simulink model "BasicAudio_TranslationEngine64"  (R2022b)
settings: Solver=FixedStepDiscrete  StartTime=0.0  StopTime=5  RelTol=1e-3  EnableMultiTasking=on
InitFcn:
  | % Initialize model
  | run([ ModelRootName() 'Init.m' ]);
  | 
  | % load library data
  | GainLibrary_data;
  | % Load saved values from partition process
  | CapturedConstMask.LoadMapFromFile(bdroot)
model workspace (MAT data in the model file):
  PreampVolumeTable_Idx = Simulink.Signal
  PreampVolumeTable_Idx.DataType = 'auto'
  PreampVolumeTable_Idx.Dimensions = -1
  PreampVolumeTable_Idx.DimensionsMode = 'auto'
  PreampVolumeTable_Idx.Complexity = 'auto'
  PreampVolumeTable_Idx.SampleTime = -1
  PreampVolumeTable_Idx.SamplingMode = 'auto'
  PreampVolumeTable_Idx.InitialValue = 'uint8([0 255 255 255 255 255])'
  Range = Simulink.Signal
  Range.DataType = 'auto'
  Range.Dimensions = -1
  Range.DimensionsMode = 'auto'
  Range.Complexity = 'auto'
  Range.SampleTime = -1
  Range.SamplingMode = 'auto'
  Table_Idx = Simulink.Signal
  Table_Idx.DataType = 'auto'
  Table_Idx.Dimensions = -1
  Table_Idx.DimensionsMode = 'auto'
  Table_Idx.Complexity = 'auto'
  Table_Idx.SampleTime = -1
  Table_Idx.SamplingMode = 'auto'
undefined symbols (not defined in the file or in its folder): Row
libraries: TuneVar x50, TOP x27, FeaturePath x7, CapturedConstLib x3
(part 1 of 4)
settings Model: Creator=kl13806
settings DataIOCC: ReturnWorkspaceOutputs=off
settings OptimizationCC: DefaultParameterBehavior=Inlined  DefaultUnderspecifiedDataType=single  EfficientTunableParamExpr=on
settings DebuggingCC: MergeDetectMultiDrivingBlocksExec=none  InheritedTsInSrcMsg=none  MultiTaskDSMMsg=none  ParameterPrecisionLossMsg=none  ParameterTunabilityLossMsg=error  UnconnectedInputMsg=warning  UnconnectedOutputMsg=warning  UnconnectedLineMsg=warning  UnknownTsInhSupMsg=none  SFUnexpectedBacktrackingDiag=warning  SFNoUnconditionalDefaultTransitionDiag=warning  SFExecutionAtInitializationDiag=none  SFMachineParentedDataDiag=warning
settings HardwareCC: ProdBitPerPointer=32  ProdBitPerSizeT=32  ProdBitPerPtrDiffT=32  ProdWordSize=32  ProdHWDeviceType=Intel->x86-32 (Windows32)  TargetBitPerPointer=64  TargetBitPerSizeT=64  TargetBitPerPtrDiffT=64  TargetLongLongMode=on  TargetIntDivRoundTo=Zero  TargetEndianess=LittleEndian  TargetWordSize=64  TargetHWDeviceType=MATLAB Host  ProdEqTarget=off
settings ModelReferenceCC: EnableRefExpFcnMdlSchedulingChecks=on  ModelReferenceNumInstancesAllowed=Single
settings SFSimCC: MATLABDynamicMemAlloc=off
settings RTWCC: Description=Embedded Coder (host-based shared library target)  SystemTargetFile=ert_shrlib.tlc  TLCOptions="-aTALARIA_ENGINE=\"Translation\""  TemplateMakefile=ert_default_tmf  RTWVerbose=off  RetainRTWFile=on  Toolchain=MinGW64 | gmake (64-bit Windows)  IncludeHyperlinkInReport=on
settings RTWCC: CustomHeaderCode=|
  | // Auto-generated code for model BasicAudio
  | /**** TOP TOKEN COMPATIBILITY HASH VALUES ****/
  | #define TOP_COMPAT {0x6E521A79UL}
  | #define TOP_COMPAT_NAME {"BasicAudio"}
  | #define TOP_COMPAT_NAME_HASH {0x9FD22631UL}
  | /**** COMPAT HASH VALUES BY MODULE ****/
  | #define BASICAUDIO_TOP_COMPAT 0x6E521A79UL
  | /**** NAME HASH VALUES BY MODULE ****/
  | #define BASICAUDIO_TOP_NAME_HASH 0x9FD22631UL
settings CodeAppCC: ForceParamTrailComments=on  IgnoreCustomStorageClasses=off  MaxIdLength=128  OperatorAnnotations=on  SimulinkDataObjDesc=on  SFDataObjDesc=on  MATLABFcnDesc=on  InsertBlockDesc=on  StateflowObjectComments=on  MATLABSourceComments=on
settings STFCustomTargetCC: TargetLangStandard=C99 (ISO)  MultiwordLength=256  ParMdlRefBuildCompliant=on  CompOptLevelCompliant=on  CombineOutputUpdateFcns=on  ERTCustomFileBanners=on  SupportContinuousTime=off  SupportNonInlinedSFcns=off  RemoveResetFunc=on  SupportVariableSizeSignals=on  MATLABClassNameForMDSCustomization=Simulink.SoftwareTarget.ERTCustomization  ModelStepFunctionPrototypeControlCompliant=on  UseToolchainInfoCompliant=on  SystemTargetFile=ert_shrlib.tlc
settings ERTTargetCC: TargetLangStandard=C99 (ISO)  ConcurrentExecutionCompliant=off  SupportVariableSizeSignals=on  CPPClassGenCompliant=off  InlinedParameterPlacement=NonHierarchical  ERTCustomFileTemplate=translation_dll.tlc  IndentStyle=Allman  IndentSize=4

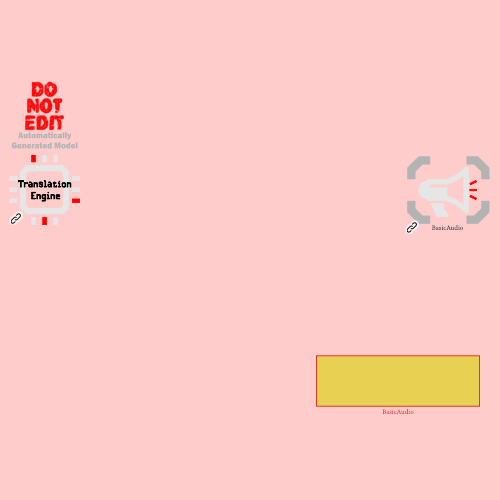
[thumbnail: Simulink's stored preview of the top-level diagram]
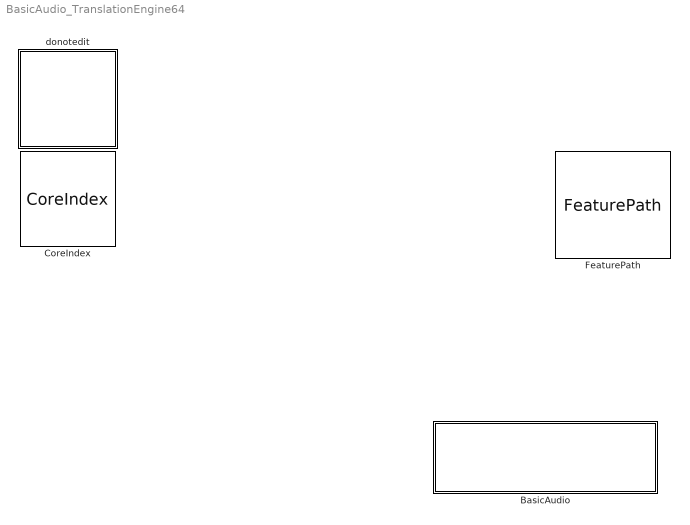
== system BasicAudio_TranslationEngine64 ==
  BasicAudio : Subsystem
  CoreIndex : FeaturePath/CoreIndex  Role=Translation Engine  CoreIndex=9  Config=[]  AddressingMode=Directly include core number in message identifiers (i.e. simple and static)  CrossCoreApi=FourListChipManager  CrossCoreAllocation=LocalCore  CrossCoreSampleTime=-1  BasePeriod=[]  TriggerInit=[-490 -501 -395 -406]
      settings: SourceProductName=Bose Talaria
  FeaturePath : FeaturePath/FeaturePath  FeatureName=BasicAudio  IsGroup=on  GroupNumber=-1  IsModule=off  TriggerInit=[45 -501 160 -394]
      settings: SourceProductName=Bose Talaria
  donotedit : Subsystem
      settings: OpenFcn=BasicAudio
      mask Display: image('DoNotEdit.svg');

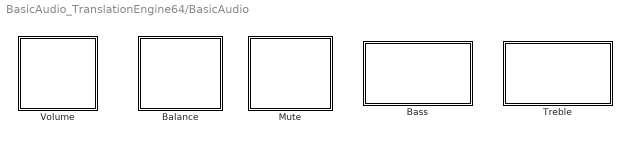
== system BasicAudio_TranslationEngine64/BasicAudio ==
  Balance : Subsystem  TreatAsAtomicUnit=on
  Bass : Subsystem  TreatAsAtomicUnit=on
  Mute : Subsystem  TreatAsAtomicUnit=on
  Treble : Subsystem  TreatAsAtomicUnit=on
  Volume : Subsystem  TreatAsAtomicUnit=on

== system BasicAudio_TranslationEngine64/donotedit ==

== system BasicAudio_TranslationEngine64/BasicAudio/Balance ==
  balance : Subsystem  mask(Bose Audio Balance){MaskFeatureName=Balance, MaskOffset=127, MaskChanRampMap=[1  2], BankNumber=0, MaskSilentExtreme=off, MaskSilentExtremeBass=on, MaskBoostDisable=off}
      mask prompts: MaskFeatureName "Feature Name (controls FeaturePath)"; MaskOffset "Control index offset"; MaskChanRampMap "Channel to Ramper map"; BankNumber "Target memory bank number:"; MaskSilentExtreme "Enable silent extreme"; MaskSilentExtremeBass "Enable silent extreme mutes bass"; MaskBoostDisable "Disable boost"
      mask help:
      | This Balance block allows for runtime control of balancing between left and right speakers/content. Based on a gain index which comes in through a control message, channel gains for 4 different content types are computed: Left, Right, Center, and Mono.
      |
      | For the Channel to Ramper Map, enter any of the following values:
      | 1 - left channel
      | 2 - right channel
      | 3 - center channel
      | 4 - mono channel
      | -1 - unused channel (will esentially be muted)
      |
      | Enable Silent Extreme if the desired outcome when accepting an index of 0 (hard left) or 255 (hard right) should completely mute the opposing channel.
      |
      | If Silent Extreme Mutes Bass is enabled, then all mono channels will be muted, when Silent Extreme is activated.
      |
      | If this block is being used in conjunction with a stand-alone Sleeping Beauty block, disable the two Silent Extreme options.
      mask init:
      | blkh = gcbh;
      | % Copy discrete mask parameters into a classdef object
      | InnerLinkConfig = BalanceConfig;
      | InnerLinkConfig.DefaultMaskOffset = MaskOffset;
      | InnerLinkConfig.DefaultMaskChanRampMap = MaskChanRampMap;
      | InnerLinkConfig.BankNumber = BankNumber;
      | InnerLinkConfig.DefaultMaskSilentExtreme = MaskSilentExtreme;
      | InnerLinkConfig.DefaultMaskSilentExtremeBass = MaskSilentExtremeBass;
      | InnerLinkConfig.DefaultMaskBoostDisable = MaskBoostDisable;
      mask Help:
      | The Balance block includes runtime control support for adjusting the balance dynamically.
      | - Channels may to be assigned to one of 4 possible rampers. Each channel needs to be assigned to a valid ramper (i.e. 1 - 4, or -1 for unused).
      | - The Index offset determines the index which corresponds to the balance being in the center position (typically 128).
      | - 'Enable silent extreme' mutes the speakers of the group whose gains are being 'cut' when at extreme indices.
      | - 'Disable boost' determines whether a boost is required or not. If selected, the maximum boost will be '1' on the linear scale ('0' in dB), otherwise he boost is calculated based on the curve (typically a maximum of 3 dB).
      | 
      | Control messages can be sent through the RTC block. The block is configured to accept a ramp time or rate (the rate has precedence) and an index which determines the gains for each channel group.
      | E.g., RTC_SIM_OBJ.AddREQ( 'BalanceSet', 0.1, [0001, <balance_index>, <ramp_db_per_second>, <ramp_milliseconds>, <subwoofer_index>, <surround_volume_index>]);
      | E.g., RTC_SIM_OBJ.AddREQ( 'BalanceSet', 0.1, [0001, 255, 0, 50, 128, 192]);
      mask TypeOptions MaskFeatureName: InnerLink/FeatureName
      mask Display:
      | [path,w,h] = IconBalanceMask();
      | 
      | % work in pixels since the icon does not scale
      | pos = get(gcbh,'position');
      | bw = pos(3) - pos(1);
      | bh = pos(4) - pos(2);
      | 
      | % Draw centered icon
      | xAdj = bw/2 - w/2;
      | yAdj = bh/2 - h/2;
      | for i=1:length(path)
      |     if (path(i).rgb(1) >= 0)
      |         patch(path(i).x+xAdj, path(i).y+yAdj, path(i).rgb);
      |     end
      |     if (path(i).stroke(1) >= 0)
      |         plot(path(i).x+xAdj, path(i).y+yAdj);
      |     end
      | end
      | 
      | % place feature name text
      | text(bw*0.5, 0, [MaskFeatureName '\n\n'], 'horizontalAlignment', 'center');

== system BasicAudio_TranslationEngine64/BasicAudio/Bass ==
  Tone : Subsystem  mask(Bose Tone High/Low){MaskFeatureName=Bass, MaskFilterType=lowpass, MaskCutHz=200, MaskCut_dB=20, MaskBoostHz=200, MaskBoost_dB=20, MaskDefaultOffset=128, MaskDefaultScale=127, BankNumber=0, TriggerInit=[90 20 195 80]}
      mask prompts: MaskFeatureName "Tone Filter Name (controls FeaturePath)"; MaskFilterType "Filter Type"; MaskCutHz "Cutoff Hz"; MaskCut_dB "Maximum dB"; MaskBoostHz "Cutoff Hz"; MaskBoost_dB "Maximum dB"; MaskDefaultOffset "Default Offset"; MaskDefaultScale "Default Scale"; BankNumber "Memory Bank Number:"; TriggerInit "Hidden: MoveFcn redraw"
      mask help: The tone block performs the treble and bass tone controls across multiple channels via a 1st order filter.
      mask init:
      | blkh = gcbh;
      | % Copy discrete mask parameters into a classdef object
      | InnerLinkConfig = ToneConfig;
      | InnerLinkConfig.FilterType = MaskFilterType;
      | InnerLinkConfig.DefaultCutHz = MaskCutHz;
      | InnerLinkConfig.DefaultCutDb = MaskCut_dB;
      | InnerLinkConfig.DefaultBoostHz = MaskBoostHz;
      | InnerLinkConfig.DefaultBoostDb = MaskBoost_dB;
      | InnerLinkConfig.DefaultOffset = MaskDefaultOffset;
      | InnerLinkConfig.DefaultScale = MaskDefaultScale;
      | InnerLinkConfig.BankNumber = BankNumber;
      settings: MoveFcn=toneMask.CB_TriggerInit(gcbh);
      mask Help:
      | The tone block performs the treble and bass tone controls across multiple channels via a 1st order filter. The treble/ bass content can either be 'boosted' or 'cut' depending on the value of the gain. Different filters can be used for the boost and cut regions, each with its own cut-off frequency.
      | 
      | MASK PARAMETERS:
      | - Different filter coefficients can be applied for the boost and cut regions
      | - The maximum boost/ cut can be specified (typically 20 dB and -20 dB)
      | - The offset and scale values determine the piecewise linear curve that maps the index to the gain (typically 128 and 127 respectively)
      | 
      | RTC CONTROL:
      | Run time control is available to dynamically change the gain to be applied to the treble/bass content. An index (typically between 0-255) can be provided along with a ramp time and rate (rate gets precedence).
      | RTC_SIM_OBJ.AddREQ( 'TrebleBassSet', 0.6, [0005,  <tone_index>, <ramp_db_per_second>, <ramp_time>]);
      | E.g., RTC_SIM_OBJ.AddREQ( 'TrebleBassSet', 0.6, [0005,  50, 0, 50]);
      mask TypeOptions MaskFeatureName: InnerLink/FeatureName
      mask TypeOptions MaskFilterType: lowpass | highpass
      mask Callback TriggerInit: ToneMask.CB_TriggerInit(gcbh);
      mask DialogControl GroupFilter Prompt: ToneFilter
      mask DialogControl GroupCut Prompt: Cut Filter
      mask DialogControl GroupBoost Prompt: Boost Filter
      mask DialogControl CalibrationGroup Prompt: Control Signal Calibration
      mask DialogControl CalibText Prompt:
      | Set the Offset and Scale to normalize the input value between -1 (maximum cut) and 1 (maximum boost) so the following equation becomes true:
      | 
      | normalized-float-value = (integer-RTC-value + Offset)  * Scale
      mask Display:
      | [path w h] = IconToneMask();
      | 
      | % retrieve the block's pixel size
      | pos = get(gcbh,'position');
      | bw = pos(3) - pos(1);
      | bh = pos(4) - pos(2);
      | 
      | % draw centered icon
      | xAdj = bw/2 - w/2;
      | yAdj = bh/2 - h/2 + 4;
      | for i=1:length(path)
      | 	patch(path(i).x+xAdj, path(i).y+yAdj, path(i).rgb);
      | end
      | 
      | % place feature name text
      | 	text(bw*0.5, 0, [MaskFeatureName '\n\n'], 'horizontalAlignment', 'center');
      | 
      | % retrieve the block's pixel size
      | pos = get(gcbh,'position');
      | bw = pos(3) - pos(1);
      | bh = pos(4) - pos(2);

== system BasicAudio_TranslationEngine64/BasicAudio/Mute ==
  mute : Subsystem  mask(Bose Audio Mute){initial_mute_state=0, MaskFeatureName=Mute, samplesPerFrame=32}
      mask prompts: initial_mute_state "Initially muted (logical)"; MaskFeatureName "Feature Name"; samplesPerFrame "Samples per frame"
      mask help: This block offers a simple mute feature using rgainy block. Set initial mute state for system cold start and a feature path name as desired. There are no tunable components, but runtime control is included.
      mask init:
      | blkh = gcbh;
      | % Copy discrete mask parameters into a classdef object
      | InnerLinkConfig = MuteConfig;
      | InnerLinkConfig.InitialMuteState = initial_mute_state;
      | InnerLinkConfig.SamplesPerFrame = samplesPerFrame;
      | 
      | % Support icon display use of ok
      | [ok,found] = MaskUtil.GetEvaluatedParameter(...
      |     MaskUtil.SubBlockName(blkh,'InnerLink'),'ok');
      | if (found == false)
      |     ok = true;
      | end
      mask Help:
      | This block offers a simple mute feature using rgainy block. The initial mute status of the block can be set through the mask.
      | 
      | RTC CONTROL:
      | Run time control is available to dynamically mute the audio. The mute status can be provided ('1' to mute audio), along with a ramp time and rate (rate gets precedence).
      | RTC_SIM_OBJ.AddREQ( 'MuteSet', 0.6, [0005,  <mute_status>, <ramp_db_per_second>, <ramp_time>]);
      | E.g., RTC_SIM_OBJ.AddREQ( 'MuteSet', 0.7, [0002, 1, 0, 50]);
      mask TypeOptions MaskFeatureName: InnerLink/FeatureName
      mask Display:
      | [path,w,h] = IconMuteMask();
      | 
      | % work in pixels since the icon does not scale
      | pos = get(gcbh,'position');
      | bw = pos(3) - pos(1);
      | bh = pos(4) - pos(2);
      | 
      | % Draw centered icon
      | xAdj = bw/2 - w/2;
      | yAdj = bh/2 - h/2;
      | for i=1:length(path)
      |     if (path(i).rgb(1) >= 0)
      |         patch(path(i).x+xAdj, path(i).y+yAdj, path(i).rgb);
      |     end
      |     if (path(i).stroke(1) >= 0)
      |         plot(path(i).x+xAdj, path(i).y+yAdj);
      |     end
      | end
      | 
      | % Display some text
      | text(bw/2, 2,MaskFeatureName, ...
      |     'horizontalAlignment','center', ...
      |     'VerticalAlignment','bottom');
      | 
      | % show a big red X when trouble is present
      | if (exist('ok','var') && ok)
      |     % Anchor the corners of the coordinate system
      |     patch(0,0,[1 1 1]);
      |     patch(bw,bh,[1 1 1]);
      | else
      |         tx=bw*0.03;
      |         ty=bh*0.03;
      |         patch([0 tx bw bw-tx], [ty 0 bh-ty bh], [1 0 0]);
      |         patch([0 bw-tx bw tx], [bh-ty 0 ty bh], [1 0 0]);
      | end

== system BasicAudio_TranslationEngine64/BasicAudio/Treble ==
  Tone : Subsystem  mask(Bose Tone High/Low){MaskFeatureName=Treble, MaskFilterType=highpass, MaskCutHz=200, MaskCut_dB=20, MaskBoostHz=200, MaskBoost_dB=20, MaskDefaultOffset=128, MaskDefaultScale=127, BankNumber=0, TriggerInit=[90 20 195 80]}
      mask prompts: MaskFeatureName "Tone Filter Name (controls FeaturePath)"; MaskFilterType "Filter Type"; MaskCutHz "Cutoff Hz"; MaskCut_dB "Maximum dB"; MaskBoostHz "Cutoff Hz"; MaskBoost_dB "Maximum dB"; MaskDefaultOffset "Default Offset"; MaskDefaultScale "Default Scale"; BankNumber "Memory Bank Number:"; TriggerInit "Hidden: MoveFcn redraw"
      mask help: The tone block performs the treble and bass tone controls across multiple channels via a 1st order filter.
      mask init: same as BasicAudio_TranslationEngine64/BasicAudio/Bass/Tone
      settings: MoveFcn=toneMask.CB_TriggerInit(gcbh);
      mask Help:
      | The tone block performs the treble and bass tone controls across multiple channels via a 1st order filter. The treble/ bass content can either be 'boosted' or 'cut' depending on the value of the gain. Different filters can be used for the boost and cut regions, each with its own cut-off frequency.
      | 
      | MASK PARAMETERS:
      | - Different filter coefficients can be applied for the boost and cut regions
      | - The maximum boost/ cut can be specified (typically 20 dB and -20 dB)
      | - The offset and scale values determine the piecewise linear curve that maps the index to the gain (typically 128 and 127 respectively)
      | 
      | RTC CONTROL:
      | Run time control is available to dynamically change the gain to be applied to the treble/bass content. An index (typically between 0-255) can be provided along with a ramp time and rate (rate gets precedence).
      | RTC_SIM_OBJ.AddREQ( 'TrebleBassSet', 0.6, [0005,  <tone_index>, <ramp_db_per_second>, <ramp_time>]);
      | E.g., RTC_SIM_OBJ.AddREQ( 'TrebleBassSet', 0.6, [0005,  50, 0, 50]);
      mask TypeOptions MaskFeatureName: InnerLink/FeatureName
      mask TypeOptions MaskFilterType: lowpass | highpass
      mask Callback TriggerInit: ToneMask.CB_TriggerInit(gcbh);
      mask DialogControl GroupFilter Prompt: ToneFilter
      mask DialogControl GroupCut Prompt: Cut Filter
      mask DialogControl GroupBoost Prompt: Boost Filter
      mask DialogControl CalibrationGroup Prompt: Control Signal Calibration
      mask DialogControl CalibText Prompt:
      | Set the Offset and Scale to normalize the input value between -1 (maximum cut) and 1 (maximum boost) so the following equation becomes true:
      | 
      | normalized-float-value = (integer-RTC-value + Offset)  * Scale
      mask Display:
      | [path w h] = IconToneMask();
      | 
      | % retrieve the block's pixel size
      | pos = get(gcbh,'position');
      | bw = pos(3) - pos(1);
      | bh = pos(4) - pos(2);
      | 
      | % draw centered icon
      | xAdj = bw/2 - w/2;
      | yAdj = bh/2 - h/2 + 4;
      | for i=1:length(path)
      | 	patch(path(i).x+xAdj, path(i).y+yAdj, path(i).rgb);
      | end
      | 
      | % place feature name text
      | 	text(bw*0.5, 0, [MaskFeatureName '\n\n'], 'horizontalAlignment', 'center');
      | 
      | % retrieve the block's pixel size
      | pos = get(gcbh,'position');
      | bw = pos(3) - pos(1);
      | bh = pos(4) - pos(2);

== system BasicAudio_TranslationEngine64/BasicAudio/Volume ==
  volume : Subsystem  mask(Bose Audio Volume){FeatureName=Volume, initial_linear_gain=0, MaskEnableGainOutput=off, MaskRows=8, MaskVolumeTable=[0 -100; 0.5 -30; 1 0], BankNumber=0, TriggerInit=[120 20 195 90]}
      mask prompts: FeatureName "Signal Name (controls FeaturePath)"; initial_linear_gain "Initial gain (linear)"; MaskEnableGainOutput "Enable output gain port"; MaskRows "Maximum Table Points"; MaskVolumeTable "Default Table"; BankNumber "Memory Bank Number:"; TriggerInit "Hidden: MoveFcn redraw"
      mask help: This volume signal block includes receipt of volume level (via RTC) as well as tuning variables to calibrate a gain table that maps 8-bit integer volume index (from RTC) to float decibels.
      mask init:
      | blkh = gcbh;
      | % Copy discrete mask parameters into a classdef object
      | InnerLinkConfig = VolumeConfig;
      | InnerLinkConfig.InitialLinearGain = initial_linear_gain;
      | InnerLinkConfig.MaskEnableGainOutput = MaskEnableGainOutput;
      | InnerLinkConfig.MaskRows = MaskRows;
      | InnerLinkConfig.MaskVolumeTable = MaskVolumeTable;
      | InnerLinkConfig.BankNumber = BankNumber;
      | 
      | % Hookup gain port
      | EnableBlockPort(blkh,'GainOut',MaskEnableGainOutput);
      settings: MoveFcn=VolumeMask.CB_TriggerInit(gcbh);
      mask Help:
      | This block allows a ramped change in volume using rgainy block.
      | - The initial gain to be applied to the input audio can be set (typically 0)
      | 
      | RTC CONTROL:
      | Run time control is available to dynamically mute the audio. The volume index can be provided (typically between 0-255), along with a ramp time and rate (rate gets precedence).
      | RTC_SIM_OBJ.AddREQ( 'VolumeSet', 0.6, [0005,  <volume_index>, <ramp_db_per_second>, <ramp_time>]);
      | E.g., RTC_SIM_OBJ.AddREQ( 'VolumeSet', 0.7, [0005, 255, 0, 50]);
      mask TypeOptions FeatureName: InnerLink/FeatureName
      mask Callback TriggerInit: VolumeMask.CB_TriggerInit(gcbh);
      mask DialogControl CalibrationGroup Prompt: Signal Calibration
      mask Display:
      | [path,w,h] = IconVolumeMask();
      | 
      | % work in pixels since the icon does not scale
      | pos = get(gcbh,'position');
      | bw = pos(3) - pos(1);
      | bh = pos(4) - pos(2);
      | 
      | % Draw centered icon
      | xAdj = bw/2 - w/2;
      | yAdj = bh/2 - h/2;
      | for i=1:length(path)
      |     if (path(i).rgb(1) >= 0)
      |         patch(path(i).x+xAdj, path(i).y+yAdj, path(i).rgb);
      |     end
      |     if (path(i).stroke(1) >= 0)
      |         plot(path(i).x+xAdj, path(i).y+yAdj);
      |     end
      | end
      | 
      | % Display some text
      | text(bw/2, bh/2,FeatureName, ...
      |     'horizontalAlignment','center', ...
      |     'VerticalAlignment','middle');

== system BasicAudio_TranslationEngine64/BasicAudio/Balance/balance ==
  InnerLink : Subsystem  mask(Blocklib Balance){FeatureName=Balance, Config=InnerLinkConfig}
      mask prompts: FeatureName "Feature path name:"; Config "BalanceConfig"
      mask help:
      | This Balance block allows for runtime control of balancing between left and right speakers/content. Based on a gain index which comes in through a control message, channel gains for 4 different content types are computed: Left, Right, Center, and Mono.
      |
      | For the Channel to Ramper Map, enter any of the following values:
      | 1 - left channel
      | 2 - right channel
      | 3 - center channel
      | 4 - mono channel
      | -1 - unused channel (will esentially be muted)
      |
      | Enable Silent Extreme if the desired outcome when accepting an index of 0 (hard left) or 255 (hard right) should completely mute the opposing channel.
      |
      | If Silent Extreme Mutes Bass is enabled, then all mono channels will be muted, when Silent Extreme is activated.
      |
      | If this block is being used in conjunction with a stand-alone Sleeping Beauty block, disable the two Silent Extreme options.
      mask init:
      | blkh=gcbh;
      | Config=BTConfig.Assert(blkh,Config);
      | 
      | BTConfig.InitSetFeatureIfPresent(blkh,'FeatureName');
      | Config.Validate();
      | 
      | % Mask init code
      | BalanceMask.Init(blkh);
      | 
      | % Flatten config for MFBs
      | MaskNumRampers = Config.NumRampers;
      | MaskBlockH = blkh;
      | % Set boundary conditions (are these supposed to be BTC?)
      | rampRateBounds = [5,50000];
      | rampTimeBounds = [1,3000];
      mask Help:
      | The Balance block includes runtime control support for adjusting the balance dynamically.
      | - Channels may to be assigned to one of 4 possible rampers. Each channel needs to be assigned to a valid ramper (i.e. 1 - 4, or -1 for unused).
      | - The Index offset determines the index which corresponds to the balance being in the center position (typically 128).
      | - 'Enable silent extreme' mutes the speakers of the group whose gains are being 'cut' when at extreme indices.
      | - 'Disable boost' determines whether a boost is required or not. If selected, the maximum boost will be '1' on the linear scale ('0' in dB), otherwise he boost is calculated based on the curve (typically a maximum of 3 dB).
      | 
      | Control messages can be sent through the RTC block. The block is configured to accept a ramp time or rate (the rate has precedence) and an index which determines the gains for each channel group.
      | E.g., RTC_SIM_OBJ.AddREQ( 'BalanceSet', 0.1, [0001, <balance_index>, <ramp_db_per_second>, <ramp_milliseconds>, <subwoofer_index>, <surround_volume_index>]);
      | E.g., RTC_SIM_OBJ.AddREQ( 'BalanceSet', 0.1, [0001, 255, 0, 50, 128, 192]);
      mask TypeOptions FeatureName: FeaturePath/FeatureName
      mask Callback Config: BTConfig.CallbackHideIfPresent(gcbh,{'FeatureName'});
      mask Display:
      | [path,w,h] = IconBalanceMask();
      | 
      | % work in pixels since the icon does not scale
      | pos = get(gcbh,'position');
      | bw = pos(3) - pos(1);
      | bh = pos(4) - pos(2);
      | 
      | % Draw centered icon
      | xAdj = bw/2 - w/2;
      | yAdj = bh/2 - h/2;
      | for i=1:length(path)
      |     if (path(i).rgb(1) >= 0)
      |         patch(path(i).x+xAdj, path(i).y+yAdj, path(i).rgb);
      |     end
      |     if (path(i).stroke(1) >= 0)
      |         plot(path(i).x+xAdj, path(i).y+yAdj);
      |     end
      | end
      | 
      | % place feature name text
      | text(bw*0.5, 0, [FeatureName '\n\n'], 'horizontalAlignment', 'center');

== system BasicAudio_TranslationEngine64/BasicAudio/Bass/Tone ==
  InnerLink : Subsystem  mask(Blocklib Tone){FeatureName=Bass, Config=InnerLinkConfig, TriggerInit=[220 160 325 220]}
      mask prompts: FeatureName "Feature path name:"; Config "ToneConfig"; TriggerInit "Hidden: MoveFcn redraw"
      mask help: The tone block performs the treble and bass tone controls across multiple channels via a 1st order filter.
      mask init:
      | blkh=gcbh;
      | Config=BTConfig.Assert(blkh,Config);
      | 
      | BTConfig.InitSetFeatureIfPresent(blkh,'FeatureName');
      | Config.Validate();
      | ToneMask.Init(blkh);
      mask Help:
      | The tone block performs the treble and bass tone controls across multiple channels via a 1st order filter. The treble/ bass content can either be 'boosted' or 'cut' depending on the value of the gain. Different filters can be used for the boost and cut regions, each with its own cut-off frequency.
      | 
      | MASK PARAMETERS:
      | - Different filter coefficients can be applied for the boost and cut regions
      | - The maximum boost/ cut can be specified (typically 20 dB and -20 dB)
      | - The offset and scale values determine the piecewise linear curve that maps the index to the gain (typically 128 and 127 respectively)
      | 
      | RTC CONTROL:
      | Run time control is available to dynamically change the gain to be applied to the treble/bass content. An index (typically between 0-255) can be provided along with a ramp time and rate (rate gets precedence).
      | RTC_SIM_OBJ.AddREQ( 'TrebleBassSet', 0.6, [0005,  <tone_index>, <ramp_db_per_second>, <ramp_time>]);
      | E.g., RTC_SIM_OBJ.AddREQ( 'TrebleBassSet', 0.6, [0005,  50, 0, 50]);
      mask TypeOptions FeatureName: FeaturePath/FeatureName
      mask Callback Config: BTConfig.CallbackHideIfPresent(gcbh,{'FeatureName'});
      mask Callback TriggerInit: ToneMask.CB_TriggerInit(gcbh);
      mask Display:
      | [path w h] = IconToneMask();
      | 
      | % retrieve the block's pixel size
      | pos = get(gcbh,'position');
      | bw = pos(3) - pos(1);
      | bh = pos(4) - pos(2);
      | 
      | % draw centered icon
      | xAdj = bw/2 - w/2;
      | yAdj = bh/2 - h/2 + 4;
      | for i=1:length(path)
      | 	patch(path(i).x+xAdj, path(i).y+yAdj, path(i).rgb);
      | end
      | 
      | % place feature name text
      | 	text(bw*0.5, 0, [FeatureName '\n\n'], 'horizontalAlignment', 'center');

== system BasicAudio_TranslationEngine64/BasicAudio/Mute/mute ==
  InnerLink : Subsystem  mask(Blocklib Mute){Config=InnerLinkConfig, FeatureName=Mute}
      mask prompts: Config "MuteConfig"; FeatureName "Mask feature name:"
      mask help: This block offers a simple mute feature using rgainy block. Set initial mute state for system cold start and a feature path name as desired. There are no tunable components, but runtime control is included.
      mask init:
      | blkh=gcbh;
      | Config=BTConfig.Assert(blkh,Config);
      | BTConfig.InitSetFeatureIfPresent(blkh,'FeatureName');
      | Config.Validate();
      mask Help:
      | This block offers a simple mute feature using rgainy block. The initial mute status of the block can be set through the mask.
      | 
      | RTC CONTROL:
      | Run time control is available to dynamically mute the audio. The mute status can be provided ('1' to mute audio), along with a ramp time and rate (rate gets precedence).
      | RTC_SIM_OBJ.AddREQ( 'MuteSet', 0.6, [0005,  <mute_status>, <ramp_db_per_second>, <ramp_time>]);
      | E.g., RTC_SIM_OBJ.AddREQ( 'MuteSet', 0.7, [0002, 1, 0, 50]);
      mask Callback Config: BTConfig.CallbackHideIfPresent(gcbh,{'FeatureName'});
      mask TypeOptions FeatureName: MuteControl/FeatureName
      mask Display:
      | [path,w,h] = IconMuteMask();
      | 
      | % work in pixels since the icon does not scale
      | pos = get(gcbh,'position');
      | bw = pos(3) - pos(1);
      | bh = pos(4) - pos(2);
      | 
      | % Draw centered icon
      | xAdj = bw/2 - w/2;
      | yAdj = bh/2 - h/2;
      | for i=1:length(path)
      |     if (path(i).rgb(1) >= 0)
      |         patch(path(i).x+xAdj, path(i).y+yAdj, path(i).rgb);
      |     end
      |     if (path(i).stroke(1) >= 0)
      |         plot(path(i).x+xAdj, path(i).y+yAdj);
      |     end
      | end
      | 
      | % Display some text
      | text(bw/2, 2,FeatureName, ...
      |     'horizontalAlignment','center', ...
      |     'VerticalAlignment','bottom');

== system BasicAudio_TranslationEngine64/BasicAudio/Treble/Tone ==
  InnerLink : Subsystem  mask(Blocklib Tone){FeatureName=Treble, Config=InnerLinkConfig, TriggerInit=[220 160 325 220]}
      mask prompts: FeatureName "Feature path name:"; Config "ToneConfig"; TriggerInit "Hidden: MoveFcn redraw"
      mask help: The tone block performs the treble and bass tone controls across multiple channels via a 1st order filter.
      mask init:
      | blkh=gcbh;
      | Config=BTConfig.Assert(blkh,Config);
      | 
      | BTConfig.InitSetFeatureIfPresent(blkh,'FeatureName');
      | Config.Validate();
      | ToneMask.Init(blkh);
      mask Help:
      | The tone block performs the treble and bass tone controls across multiple channels via a 1st order filter. The treble/ bass content can either be 'boosted' or 'cut' depending on the value of the gain. Different filters can be used for the boost and cut regions, each with its own cut-off frequency.
      | 
      | MASK PARAMETERS:
      | - Different filter coefficients can be applied for the boost and cut regions
      | - The maximum boost/ cut can be specified (typically 20 dB and -20 dB)
      | - The offset and scale values determine the piecewise linear curve that maps the index to the gain (typically 128 and 127 respectively)
      | 
      | RTC CONTROL:
      | Run time control is available to dynamically change the gain to be applied to the treble/bass content. An index (typically between 0-255) can be provided along with a ramp time and rate (rate gets precedence).
      | RTC_SIM_OBJ.AddREQ( 'TrebleBassSet', 0.6, [0005,  <tone_index>, <ramp_db_per_second>, <ramp_time>]);
      | E.g., RTC_SIM_OBJ.AddREQ( 'TrebleBassSet', 0.6, [0005,  50, 0, 50]);
      mask TypeOptions FeatureName: FeaturePath/FeatureName
      mask Callback Config: BTConfig.CallbackHideIfPresent(gcbh,{'FeatureName'});
      mask Callback TriggerInit: ToneMask.CB_TriggerInit(gcbh);
      mask Display:
      | [path w h] = IconToneMask();
      | 
      | % retrieve the block's pixel size
      | pos = get(gcbh,'position');
      | bw = pos(3) - pos(1);
      | bh = pos(4) - pos(2);
      | 
      | % draw centered icon
      | xAdj = bw/2 - w/2;
      | yAdj = bh/2 - h/2 + 4;
      | for i=1:length(path)
      | 	patch(path(i).x+xAdj, path(i).y+yAdj, path(i).rgb);
      | end
      | 
      | % place feature name text
      | 	text(bw*0.5, 0, [FeatureName '\n\n'], 'horizontalAlignment', 'center');

== system BasicAudio_TranslationEngine64/BasicAudio/Volume/volume ==
  InnerLink : Subsystem  mask(Blocklib Volume){FeatureName=Volume, Config=InnerLinkConfig, EnableGainOut=on, TriggerInit=[60 35 135 110]}
      mask prompts: FeatureName "Feature path name:"; Config "VolumeConfig"; EnableGainOut "Enable gain output"; TriggerInit "Hidden: MoveFcn redraw"
      mask help: This volume signal block includes receipt of volume level (via RTC) as well as tuning variables to calibrate a gain table that maps 8-bit integer volume index (from RTC) to float decibels.
      mask init:
      | blkh=gcbh;
      | Config=BTConfig.Assert(blkh,Config);
      | 
      | % Set boundary conditions
      | rampRateBounds = [5,50000];
      | rampTimeBounds = [1,3000];
      | BTConfig.InitSetFeatureIfPresent(blkh,'FeatureName');
      | Config.Validate();
      | 
      | EnableBlockPort(blkh,'gain out',EnableGainOut);
      settings: MoveFcn=VolumeMask.CB_TriggerInit(gcbh);
      mask Help:
      | This block allows a ramped change in volume using rgainy block.
      | - The initial gain to be applied to the input audio can be set (typically 0)
      | 
      | RTC CONTROL:
      | Run time control is available to dynamically mute the audio. The volume index can be provided (typically between 0-255), along with a ramp time and rate (rate gets precedence).
      | RTC_SIM_OBJ.AddREQ( 'VolumeSet', 0.6, [0005,  <volume_index>, <ramp_db_per_second>, <ramp_time>]);
      | E.g., RTC_SIM_OBJ.AddREQ( 'VolumeSet', 0.7, [0005, 255, 0, 50]);
      mask TypeOptions FeatureName: FeaturePath/FeatureName
      mask Callback Config: BTConfig.CallbackHideIfPresent(gcbh,{'FeatureName'});
      mask Callback TriggerInit: VolumeMask.CB_TriggerInit(gcbh);
      mask Display:
      | [path,w,h] = IconVolumeMask();
      | 
      | % work in pixels since the icon does not scale
      | pos = get(gcbh,'position');
      | bw = pos(3) - pos(1);
      | bh = pos(4) - pos(2);
      | 
      | % Draw centered icon
      | xAdj = bw/2 - w/2;
      | yAdj = bh/2 - h/2;
      | for i=1:length(path)
      |     if (path(i).rgb(1) >= 0)
      |         patch(path(i).x+xAdj, path(i).y+yAdj, path(i).rgb);
      |     end
      |     if (path(i).stroke(1) >= 0)
      |         plot(path(i).x+xAdj, path(i).y+yAdj);
      |     end
      | end
      | 
      | % Display some text
      | text(bw/2, bh/2,FeatureName, ...
      |     'horizontalAlignment','center', ...
      |     'VerticalAlignment','middle');
